simulink model "EV_Modeling_old"  (R2024b)
settings: Solver=FixedStepAuto  StartTime=0.0  StopTime=10382  FixedStep=0.1  RelTol=1e-3
values from neighbouring files (symbols this model uses):
  battery_SOC_SOC = battery_SOC(:,1)    [EV_Truck.m]    (also in simulink.m)
  battery_SOC_voltage = battery_SOC(:,2)    [EV_Truck.m]    (also in simulink.m)
  drag_coefficient_FV1 = table2array(drag_coefficient(:,3))    [simulink.m]
  drag_coefficient_FV2 = table2array(drag_coefficient(:,4))    [simulink.m]
  drag_coefficient_input = table2array(drag_coefficient(:,1))    [simulink.m]
  drag_coefficient_LV = table2array(drag_coefficient(:,2))    [simulink.m]
  electric_consumption_ressistancce = electric_consumption(:,2)    [EV_Truck.m]    (also in simulink.m)
  electric_consumption_voltage = electric_consumption(:,1)    [EV_Truck.m]    (also in simulink.m)
  motor_efficiency_efficiency = table2array(motor_efficiency(2:height(motor_efficiency),2:width(motor_efficiency)))    [EV_Truck.m]    (also in simulink.m)
  motor_efficiency_RPM = table2array(motor_efficiency(2:height(motor_efficiency),1))    [EV_Truck.m]    (also in simulink.m)
  motor_efficiency_torque = transpose(motor_efficiency_torque)    [EV_Truck.m]    (also in simulink.m)
  motor_RPM_torque = table2array(motor_torque(1:14,1))    [EV_Truck.m]    (also in simulink.m)
  motor_torque_RPM = table2array(motor_torque(1:14,2))    [EV_Truck.m]    (also in simulink.m)
undefined symbols (not defined in the file or in its folder): battery_builder_rtmsupport, battery_sli_rtmsupport, C1_mat, C2_mat, c_sqrt, DiscIntNeverNeededParam, dV0_mat, gcbh, n, Wc, Wm, x0
libraries: simulink x87, packLibrary_lib x30, nesl_utility x6, fl_lib x6, simulink_extras x3, mpcadaslib x2, slpidlib x1
(part 7 of 12)

== system EV_Modeling_old/LV/SOC Estimator (Kalman Filter)/Kalman Filter/UKBF 2RC ==
  CellVoltage : Inport
  Current : Inport  Port=2
  CellTemperature : Inport  Port=3
  InitialSOC : Inport  Port=4
  Constant : Constant  Value=chol(P0_2RC,'lower')
  Constant1 : Constant  Value=0  VectorParams1D=off
  Data Type Conversion{,1..3} (4 alike) : DataTypeConversion  OutDataTypeStr=double  SaturateOnIntegerOverflow=off  RndMeth=Floor
  Mux : Mux  Inputs=3
  Prediction-correction : Subsystem
  Reshape : Reshape  OutputDimensionality=Customize  OutputDimensions=[n,1]
  Reshape1 : Reshape
  Sigma points init : Subsystem
  xhat : Outport
  wires:
  Data Type Conversion/1 -> Prediction-correction/1(Current)
  Data Type Conversion3/1 -> Mux/1
  Data Type Conversion2/1 -> Prediction-correction/3(Voltage)
  Reshape/1 -> Sigma points init/1(x0)
  InitialSOC/1 -> Data Type Conversion3/1
  Constant/1 -> Sigma points init/2(A)
  Data Type Conversion1/1 -> Prediction-correction/2(Temperature)
  Constant1/1 -> Mux/3, Mux/2
  Prediction-correction/1(xhat) -> Reshape1/1
  Sigma points init/1(X0) -> Prediction-correction/4(X0)
  CellTemperature/1 -> Data Type Conversion1/1
  CellVoltage/1 -> Data Type Conversion2/1
  Mux/1 -> Reshape/1
  Current/1 -> Data Type Conversion/1
  Reshape1/1 -> xhat/1

== system EV_Modeling_old/LV/SOC Estimator (Kalman Filter)/Kalman Filter/UKF ==
  CellVoltage : Inport
  Current : Inport  Port=2
  CellTemperature : Inport  Port=3
  InitialSOC : Inport  Port=4
  Correction : Subsystem
  Delay - X : Subsystem
      settings: PortSchema="{\"entries\":[{\"content\":{\"sides\":[{\"content\":{\"connectorIds\":[\"In1\"]},\"type\":\"ConnectorPlacement.EquallySpacedRectSide\",\"uuid\":\"3362b6e3-9ef0-414f-8c36-2f543f704d9c\"},{\"content\":{\"connectorIds\":[\"Out1\",\"In2\"],\"side\":\"RIGHT\"},\"type\":\"ConnectorPlacement.EquallySpacedRectSide\",\"uuid\":\"11e7d0c5-4a27-4b8c-b505-ab30596c2b25\"},{\"content\":{\"connectorIds\":[],\"side\":\"TOP\"},\"type\":\"ConnectorPlacement.EquallySpacedRectSide\",\"uuid\":\"2d2b4d79-d4b9-4064-9377-c3a75a280e90\"}]},\"type\":\"ConnectorPlacement.EquallySpacedConnector\",\"uuid\":\"61e54eb8-002c-4ced-aad8-a34ad65d09af\"}],\"packageUris\":[\"http://schema.mathworks.com/mf0/Connector/R2020b\"],\"version\":\"1.0\"}"
  Prediction : Subsystem
  Rate Transition{,1..3} (4 alike) : RateTransition  OutPortSampleTime=Ts
  Reshape : Reshape
  Sigma points : Subsystem
  Sum : Sum  Inputs=+-|
  Unit Delay - P : UnitDelay  InitialCondition=chol(P0,'lower')  SampleTime=Ts  HasFrameUpgradeWarning=on
  xhat : Outport
  wires:
  Prediction/1(Yk1_k) -> Sum/2
  CellVoltage/1 -> Rate Transition/1
  Prediction/5(Pk1k) -> Correction/5(Pk1_k)
  Current/1 -> Rate Transition1/1
  Delay - X/1(y) -> Sigma points/1(x)
  Sum/1 -> Correction/1(Vt_error)
  Sigma points/1(X) -> Prediction/3(X)
  CellTemperature/1 -> Rate Transition2/1
  Prediction/4(Py) -> Correction/4(Py)
  Prediction/3(Pxy) -> Correction/3(Pxy)
  Unit Delay - P/1 -> Sigma points/2(P)
  Correction/1(xk1_k1) -> Delay - X/1(u), Reshape/1
  Correction/2(Pk1_k1) -> Unit Delay - P/1
  Prediction/2(Xk1_k) -> Correction/2(xk1_k)
  Reshape/1 -> xhat/1
  Rate Transition/1 -> Sum/1
  Rate Transition1/1 -> Prediction/1(Current)
  Rate Transition2/1 -> Prediction/2(Temperature)
  InitialSOC/1 -> Rate Transition3/1
  Rate Transition3/1 -> Delay - X/2(SOC0)

== system EV_Modeling_old/LV/SOC Estimator (Kalman Filter)/Kalman Filter/UKF 2RC ==
  CellVoltage : Inport
  Current : Inport  Port=2
  CellTemperature : Inport  Port=3
  InitialSOC : Inport  Port=4
  Correction : Subsystem
  Delay - X : Subsystem
      settings: PortSchema="{\"entries\":[{\"content\":{\"sides\":[{\"content\":{\"connectorIds\":[\"In1\"]},\"type\":\"ConnectorPlacement.EquallySpacedRectSide\",\"uuid\":\"3362b6e3-9ef0-414f-8c36-2f543f704d9c\"},{\"content\":{\"connectorIds\":[\"Out1\",\"In2\"],\"side\":\"RIGHT\"},\"type\":\"ConnectorPlacement.EquallySpacedRectSide\",\"uuid\":\"11e7d0c5-4a27-4b8c-b505-ab30596c2b25\"},{\"content\":{\"connectorIds\":[],\"side\":\"TOP\"},\"type\":\"ConnectorPlacement.EquallySpacedRectSide\",\"uuid\":\"2d2b4d79-d4b9-4064-9377-c3a75a280e90\"}]},\"type\":\"ConnectorPlacement.EquallySpacedConnector\",\"uuid\":\"61e54eb8-002c-4ced-aad8-a34ad65d09af\"}],\"packageUris\":[\"http://schema.mathworks.com/mf0/Connector/R2020b\"],\"version\":\"1.0\"}"
  Prediction : Subsystem
  Rate Transition{,1..3} (4 alike) : RateTransition  OutPortSampleTime=Ts
  Reshape : Reshape
  Sigma points : Subsystem
  Sum : Sum  Inputs=+-|
  Unit Delay - P : UnitDelay  InitialCondition=chol(P0_2RC,'lower')  SampleTime=Ts  HasFrameUpgradeWarning=on
  xhat : Outport
  wires:
  Rate Transition/1 -> Sum/1
  Rate Transition3/1 -> Delay - X/2(SOC0)
  CellTemperature/1 -> Rate Transition2/1
  Correction/1(xk1_k1) -> Delay - X/1(u), Reshape/1
  Prediction/2(Xk1_k) -> Correction/2(xk1_k)
  InitialSOC/1 -> Rate Transition3/1
  Unit Delay - P/1 -> Sigma points/2(P)
  Current/1 -> Rate Transition1/1
  Prediction/1(Yk1_k) -> Sum/2
  Rate Transition1/1 -> Prediction/1(Current)
  Rate Transition2/1 -> Prediction/2(Temperature)
  Sum/1 -> Correction/1(Vt_error)
  Prediction/5(Pk1k) -> Correction/5(Pk1_k)
  Prediction/4(Py) -> Correction/4(Py)
  Prediction/3(Pxy) -> Correction/3(Pxy)
  Sigma points/1(X) -> Prediction/3(X)
  Reshape/1 -> xhat/1
  CellVoltage/1 -> Rate Transition/1
  Correction/2(Pk1_k1) -> Unit Delay - P/1
  Delay - X/1(y) -> Sigma points/1(x)

== system EV_Modeling_old/LV/Subsystem/Pack1/ModuleAssembly1 ==
  note: Battery Modules
  note: Output Signals
  Module1 : packLibrary_lib/Modules/ModuleType1  SOC_vecCell=[0, .1, .25, .5, .75, .9, 1]  V0_vecCell=[3.5057, 3.566, 3.6337, 3.7127, 3.9259, 4.0777, 4.1928] V  V_rangeCell=[0, inf] V  R0_vecCell=[.0085, .0085, .0087, .0082, .0083, .0085, .0085] Ohm  AHCell=5 Ah  extrapolation_optionCell=simscape.enum.extrapolation.nearest  P=3  S=11  iCell_specify=off  iCell_priority=None  iCell=0 A  iCell_nominal_specify=off  iCell_nominal_value=1  iCell_nominal_unit=A  vCell_specify=off  vCell_priority=None  vCell=0 V  vCell_nominal_specify=off  vCell_nominal_value=1  vCell_nominal_unit=V  socCell_specify=off  socCell_priority=High  socCell=1  socCell_nominal_specify=off  socCell_nominal_value=1  socCell_nominal_unit=1  numCyclesCell_specify=off  numCyclesCell_priority=High  numCyclesCell=0  numCyclesCell_nominal_specify=off  numCyclesCell_nominal_value=1  numCyclesCell_nominal_unit=1  vParallelAssembly_specify=off  vParallelAssembly_priority=None  vParallelAssembly=repmat(0, 11, 1) V  vParallelAssembly_nominal_specify=off  vParallelAssembly_nominal_value=1  vParallelAssembly_nominal_unit=V  socParallelAssembly_specify=off  socParallelAssembly_priority=None  socParallelAssembly=repmat(1, 11, 1)  socParallelAssembly_nominal_specify=off  socParallelAssembly_nominal_value=1  socParallelAssembly_nominal_unit=1
      settings: InternalSimscapePortConfiguration="{\"Bottom\":[{\"id\":\"n\",\"label\":\"-\",\"type\":\"foundation.electrical.electrical\"}],\"Left\":[],\"Right\":[],\"Top\":[{\"id\":\"p\",\"label\":\"+\",\"type\":\"foundation.electrical.electrical\"}]}"
  Module1_outputs : SimscapeProbe  BoundBlock=553  Variables="{\"iCell\":{\"Unit\":\"A\",\"PortLabel\":\"iCell\",\"Probing\":\"ON\"},\"numCyclesCell\":{\"Unit\":\"1\",\"PortLabel\":\"numCyclesCell\",\"Probing\":\"ON\"},\"socCell\":{\"Unit\":\"1\",\"PortLabel\":\"socCell\",\"Probing\":\"ON\"},\"socParallelAssembly\":{\"Unit\":\"1\",\"PortLabel\":\"socParallelAssembly\",\"Probing\":\"ON\"},\"vCell\":{\"Unit\":\"V\",\"PortLabel\":\"vCell\",\"Probing\":\"ON\"},\"vParallelAssembly\":{\"Unit\":\"V\",\"PortLabel\":\"vParallelAssembly\",\"Probing\":\"ON\"}}"
  Module2 : packLibrary_lib/Modules/ModuleType1  SOC_vecCell=[0, .1, .25, .5, .75, .9, 1]  V0_vecCell=[3.5057, 3.566, 3.6337, 3.7127, 3.9259, 4.0777, 4.1928] V  V_rangeCell=[0, inf] V  R0_vecCell=[.0085, .0085, .0087, .0082, .0083, .0085, .0085] Ohm  AHCell=5 Ah  extrapolation_optionCell=simscape.enum.extrapolation.nearest  P=3  S=11  iCell_specify=off  iCell_priority=None  iCell=0 A  iCell_nominal_specify=off  iCell_nominal_value=1  iCell_nominal_unit=A  vCell_specify=off  vCell_priority=None  vCell=0 V  vCell_nominal_specify=off  vCell_nominal_value=1  vCell_nominal_unit=V  socCell_specify=off  socCell_priority=High  socCell=1  socCell_nominal_specify=off  socCell_nominal_value=1  socCell_nominal_unit=1  numCyclesCell_specify=off  numCyclesCell_priority=High  numCyclesCell=0  numCyclesCell_nominal_specify=off  numCyclesCell_nominal_value=1  numCyclesCell_nominal_unit=1  vParallelAssembly_specify=off  vParallelAssembly_priority=None  vParallelAssembly=repmat(0, 11, 1) V  vParallelAssembly_nominal_specify=off  vParallelAssembly_nominal_value=1  vParallelAssembly_nominal_unit=V  socParallelAssembly_specify=off  socParallelAssembly_priority=None  socParallelAssembly=repmat(1, 11, 1)  socParallelAssembly_nominal_specify=off  socParallelAssembly_nominal_value=1  socParallelAssembly_nominal_unit=1
      settings: InternalSimscapePortConfiguration="{\"Bottom\":[{\"id\":\"n\",\"label\":\"-\",\"type\":\"foundation.electrical.electrical\"}],\"Left\":[],\"Right\":[],\"Top\":[{\"id\":\"p\",\"label\":\"+\",\"type\":\"foundation.electrical.electrical\"}]}"
  Module2_outputs : SimscapeProbe  BoundBlock=555  Variables="{\"iCell\":{\"Unit\":\"A\",\"PortLabel\":\"iCell\",\"Probing\":\"ON\"},\"numCyclesCell\":{\"Unit\":\"1\",\"PortLabel\":\"numCyclesCell\",\"Probing\":\"ON\"},\"socCell\":{\"Unit\":\"1\",\"PortLabel\":\"socCell\",\"Probing\":\"ON\"},\"socParallelAssembly\":{\"Unit\":\"1\",\"PortLabel\":\"socParallelAssembly\",\"Probing\":\"ON\"},\"vCell\":{\"Unit\":\"V\",\"PortLabel\":\"vCell\",\"Probing\":\"ON\"},\"vParallelAssembly\":{\"Unit\":\"V\",\"PortLabel\":\"vParallelAssembly\",\"Probing\":\"ON\"}}"
  iCellMux : Mux  Inputs=2
  numCyclesCellMux : Mux  Inputs=2
  socCellMux : Mux  Inputs=2
  socParallelAssemblyMux : Mux  Inputs=2
  vCellMux : Mux  Inputs=2
  vParallelAssemblyMux : Mux  Inputs=2
  + : PMIOPort  Side=Left
  - : PMIOPort  Port=2  Side=Right
  iCell : Outport
  numCyclesCell : Outport  Port=2
  socCell : Outport  Port=3
  socParallelAssembly : Outport  Port=4
  vCell : Outport  Port=5
  vParallelAssembly : Outport  Port=6
  wires:
  Module1_outputs/1 -> [iCell1]
  iCellMux/1 -> iCell/1
  [iCell1] -> iCellMux/1
  Module1_outputs/2 -> [numCyclesCell1]
  numCyclesCellMux/1 -> numCyclesCell/1
  [numCyclesCell1] -> numCyclesCellMux/1
  Module1_outputs/3 -> [socCell1]
  socCellMux/1 -> socCell/1
  [socCell1] -> socCellMux/1
  Module1_outputs/4 -> [socParallelAssembly1]
  socParallelAssemblyMux/1 -> socParallelAssembly/1
  [socParallelAssembly1] -> socParallelAssemblyMux/1
  Module1_outputs/5 -> [vCell1]
  vCellMux/1 -> vCell/1
  [vCell1] -> vCellMux/1
  Module1_outputs/6 -> [vParallelAssembly1]
  vParallelAssemblyMux/1 -> vParallelAssembly/1
  [vParallelAssembly1] -> vParallelAssemblyMux/1
  Module2_outputs/1 -> [iCell2]
  [iCell2] -> iCellMux/2
  Module2_outputs/2 -> [numCyclesCell2]
  [numCyclesCell2] -> numCyclesCellMux/2
  Module2_outputs/3 -> [socCell2]
  [socCell2] -> socCellMux/2
  Module2_outputs/4 -> [socParallelAssembly2]
  [socParallelAssembly2] -> socParallelAssemblyMux/2
  Module2_outputs/5 -> [vCell2]
  [vCell2] -> vCellMux/2
  Module2_outputs/6 -> [vParallelAssembly2]
  [vParallelAssembly2] -> vParallelAssemblyMux/2
  connections:
  Module2/LConn1 -- Module1/RConn1
  Module1/LConn1 -- +/RConn1
  Module2/RConn1 -- -/RConn1

== system EV_Modeling_old/LV/Subsystem/Pack1/ModuleAssembly2 ==
  note: Battery Modules
  note: Output Signals
  Module1 : packLibrary_lib/Modules/ModuleType1  SOC_vecCell=[0, .1, .25, .5, .75, .9, 1]  V0_vecCell=[3.5057, 3.566, 3.6337, 3.7127, 3.9259, 4.0777, 4.1928] V  V_rangeCell=[0, inf] V  R0_vecCell=[.0085, .0085, .0087, .0082, .0083, .0085, .0085] Ohm  AHCell=5 Ah  extrapolation_optionCell=simscape.enum.extrapolation.nearest  P=3  S=11  iCell_specify=off  iCell_priority=None  iCell=0 A  iCell_nominal_specify=off  iCell_nominal_value=1  iCell_nominal_unit=A  vCell_specify=off  vCell_priority=None  vCell=0 V  vCell_nominal_specify=off  vCell_nominal_value=1  vCell_nominal_unit=V  socCell_specify=off  socCell_priority=High  socCell=1  socCell_nominal_specify=off  socCell_nominal_value=1  socCell_nominal_unit=1  numCyclesCell_specify=off  numCyclesCell_priority=High  numCyclesCell=0  numCyclesCell_nominal_specify=off  numCyclesCell_nominal_value=1  numCyclesCell_nominal_unit=1  vParallelAssembly_specify=off  vParallelAssembly_priority=None  vParallelAssembly=repmat(0, 11, 1) V  vParallelAssembly_nominal_specify=off  vParallelAssembly_nominal_value=1  vParallelAssembly_nominal_unit=V  socParallelAssembly_specify=off  socParallelAssembly_priority=None  socParallelAssembly=repmat(1, 11, 1)  socParallelAssembly_nominal_specify=off  socParallelAssembly_nominal_value=1  socParallelAssembly_nominal_unit=1
      settings: InternalSimscapePortConfiguration="{\"Bottom\":[{\"id\":\"n\",\"label\":\"-\",\"type\":\"foundation.electrical.electrical\"}],\"Left\":[],\"Right\":[],\"Top\":[{\"id\":\"p\",\"label\":\"+\",\"type\":\"foundation.electrical.electrical\"}]}"
  Module1_outputs : SimscapeProbe  BoundBlock=598  Variables="{\"iCell\":{\"Unit\":\"A\",\"PortLabel\":\"iCell\",\"Probing\":\"ON\"},\"numCyclesCell\":{\"Unit\":\"1\",\"PortLabel\":\"numCyclesCell\",\"Probing\":\"ON\"},\"socCell\":{\"Unit\":\"1\",\"PortLabel\":\"socCell\",\"Probing\":\"ON\"},\"socParallelAssembly\":{\"Unit\":\"1\",\"PortLabel\":\"socParallelAssembly\",\"Probing\":\"ON\"},\"vCell\":{\"Unit\":\"V\",\"PortLabel\":\"vCell\",\"Probing\":\"ON\"},\"vParallelAssembly\":{\"Unit\":\"V\",\"PortLabel\":\"vParallelAssembly\",\"Probing\":\"ON\"}}"
  Module2 : packLibrary_lib/Modules/ModuleType1  SOC_vecCell=[0, .1, .25, .5, .75, .9, 1]  V0_vecCell=[3.5057, 3.566, 3.6337, 3.7127, 3.9259, 4.0777, 4.1928] V  V_rangeCell=[0, inf] V  R0_vecCell=[.0085, .0085, .0087, .0082, .0083, .0085, .0085] Ohm  AHCell=5 Ah  extrapolation_optionCell=simscape.enum.extrapolation.nearest  P=3  S=11  iCell_specify=off  iCell_priority=None  iCell=0 A  iCell_nominal_specify=off  iCell_nominal_value=1  iCell_nominal_unit=A  vCell_specify=off  vCell_priority=None  vCell=0 V  vCell_nominal_specify=off  vCell_nominal_value=1  vCell_nominal_unit=V  socCell_specify=off  socCell_priority=High  socCell=1  socCell_nominal_specify=off  socCell_nominal_value=1  socCell_nominal_unit=1  numCyclesCell_specify=off  numCyclesCell_priority=High  numCyclesCell=0  numCyclesCell_nominal_specify=off  numCyclesCell_nominal_value=1  numCyclesCell_nominal_unit=1  vParallelAssembly_specify=off  vParallelAssembly_priority=None  vParallelAssembly=repmat(0, 11, 1) V  vParallelAssembly_nominal_specify=off  vParallelAssembly_nominal_value=1  vParallelAssembly_nominal_unit=V  socParallelAssembly_specify=off  socParallelAssembly_priority=None  socParallelAssembly=repmat(1, 11, 1)  socParallelAssembly_nominal_specify=off  socParallelAssembly_nominal_value=1  socParallelAssembly_nominal_unit=1
      settings: InternalSimscapePortConfiguration="{\"Bottom\":[{\"id\":\"n\",\"label\":\"-\",\"type\":\"foundation.electrical.electrical\"}],\"Left\":[],\"Right\":[],\"Top\":[{\"id\":\"p\",\"label\":\"+\",\"type\":\"foundation.electrical.electrical\"}]}"
  Module2_outputs : SimscapeProbe  BoundBlock=600  Variables="{\"iCell\":{\"Unit\":\"A\",\"PortLabel\":\"iCell\",\"Probing\":\"ON\"},\"numCyclesCell\":{\"Unit\":\"1\",\"PortLabel\":\"numCyclesCell\",\"Probing\":\"ON\"},\"socCell\":{\"Unit\":\"1\",\"PortLabel\":\"socCell\",\"Probing\":\"ON\"},\"socParallelAssembly\":{\"Unit\":\"1\",\"PortLabel\":\"socParallelAssembly\",\"Probing\":\"ON\"},\"vCell\":{\"Unit\":\"V\",\"PortLabel\":\"vCell\",\"Probing\":\"ON\"},\"vParallelAssembly\":{\"Unit\":\"V\",\"PortLabel\":\"vParallelAssembly\",\"Probing\":\"ON\"}}"
  iCellMux : Mux  Inputs=2
  numCyclesCellMux : Mux  Inputs=2
  socCellMux : Mux  Inputs=2
  socParallelAssemblyMux : Mux  Inputs=2
  vCellMux : Mux  Inputs=2
  vParallelAssemblyMux : Mux  Inputs=2
  + : PMIOPort  Side=Left
  - : PMIOPort  Port=2  Side=Right
  iCell : Outport
  numCyclesCell : Outport  Port=2
  socCell : Outport  Port=3
  socParallelAssembly : Outport  Port=4
  vCell : Outport  Port=5
  vParallelAssembly : Outport  Port=6
  wires:
  Module1_outputs/1 -> [iCell1]
  iCellMux/1 -> iCell/1
  [iCell1] -> iCellMux/1
  Module1_outputs/2 -> [numCyclesCell1]
  numCyclesCellMux/1 -> numCyclesCell/1
  [numCyclesCell1] -> numCyclesCellMux/1
  Module1_outputs/3 -> [socCell1]
  socCellMux/1 -> socCell/1
  [socCell1] -> socCellMux/1
  Module1_outputs/4 -> [socParallelAssembly1]
  socParallelAssemblyMux/1 -> socParallelAssembly/1
  [socParallelAssembly1] -> socParallelAssemblyMux/1
  Module1_outputs/5 -> [vCell1]
  vCellMux/1 -> vCell/1
  [vCell1] -> vCellMux/1
  Module1_outputs/6 -> [vParallelAssembly1]
  vParallelAssemblyMux/1 -> vParallelAssembly/1
  [vParallelAssembly1] -> vParallelAssemblyMux/1
  Module2_outputs/1 -> [iCell2]
  [iCell2] -> iCellMux/2
  Module2_outputs/2 -> [numCyclesCell2]
  [numCyclesCell2] -> numCyclesCellMux/2
  Module2_outputs/3 -> [socCell2]
  [socCell2] -> socCellMux/2
  Module2_outputs/4 -> [socParallelAssembly2]
  [socParallelAssembly2] -> socParallelAssemblyMux/2
  Module2_outputs/5 -> [vCell2]
  [vCell2] -> vCellMux/2
  Module2_outputs/6 -> [vParallelAssembly2]
  [vParallelAssembly2] -> vParallelAssemblyMux/2
  connections:
  Module2/LConn1 -- Module1/RConn1
  Module1/LConn1 -- +/RConn1
  Module2/RConn1 -- -/RConn1

== system EV_Modeling_old/LV/Subsystem/Pack1/ModuleAssembly3 ==
  note: Battery Modules
  note: Output Signals
  Module1 : packLibrary_lib/Modules/ModuleType1  SOC_vecCell=[0, .1, .25, .5, .75, .9, 1]  V0_vecCell=[3.5057, 3.566, 3.6337, 3.7127, 3.9259, 4.0777, 4.1928] V  V_rangeCell=[0, inf] V  R0_vecCell=[.0085, .0085, .0087, .0082, .0083, .0085, .0085] Ohm  AHCell=5 Ah  extrapolation_optionCell=simscape.enum.extrapolation.nearest  P=3  S=11  iCell_specify=off  iCell_priority=None  iCell=0 A  iCell_nominal_specify=off  iCell_nominal_value=1  iCell_nominal_unit=A  vCell_specify=off  vCell_priority=None  vCell=0 V  vCell_nominal_specify=off  vCell_nominal_value=1  vCell_nominal_unit=V  socCell_specify=off  socCell_priority=High  socCell=1  socCell_nominal_specify=off  socCell_nominal_value=1  socCell_nominal_unit=1  numCyclesCell_specify=off  numCyclesCell_priority=High  numCyclesCell=0  numCyclesCell_nominal_specify=off  numCyclesCell_nominal_value=1  numCyclesCell_nominal_unit=1  vParallelAssembly_specify=off  vParallelAssembly_priority=None  vParallelAssembly=repmat(0, 11, 1) V  vParallelAssembly_nominal_specify=off  vParallelAssembly_nominal_value=1  vParallelAssembly_nominal_unit=V  socParallelAssembly_specify=off  socParallelAssembly_priority=None  socParallelAssembly=repmat(1, 11, 1)  socParallelAssembly_nominal_specify=off  socParallelAssembly_nominal_value=1  socParallelAssembly_nominal_unit=1
      settings: InternalSimscapePortConfiguration="{\"Bottom\":[{\"id\":\"n\",\"label\":\"-\",\"type\":\"foundation.electrical.electrical\"}],\"Left\":[],\"Right\":[],\"Top\":[{\"id\":\"p\",\"label\":\"+\",\"type\":\"foundation.electrical.electrical\"}]}"
  Module1_outputs : SimscapeProbe  BoundBlock=643  Variables="{\"iCell\":{\"Unit\":\"A\",\"PortLabel\":\"iCell\",\"Probing\":\"ON\"},\"numCyclesCell\":{\"Unit\":\"1\",\"PortLabel\":\"numCyclesCell\",\"Probing\":\"ON\"},\"socCell\":{\"Unit\":\"1\",\"PortLabel\":\"socCell\",\"Probing\":\"ON\"},\"socParallelAssembly\":{\"Unit\":\"1\",\"PortLabel\":\"socParallelAssembly\",\"Probing\":\"ON\"},\"vCell\":{\"Unit\":\"V\",\"PortLabel\":\"vCell\",\"Probing\":\"ON\"},\"vParallelAssembly\":{\"Unit\":\"V\",\"PortLabel\":\"vParallelAssembly\",\"Probing\":\"ON\"}}"
  Module2 : packLibrary_lib/Modules/ModuleType1  SOC_vecCell=[0, .1, .25, .5, .75, .9, 1]  V0_vecCell=[3.5057, 3.566, 3.6337, 3.7127, 3.9259, 4.0777, 4.1928] V  V_rangeCell=[0, inf] V  R0_vecCell=[.0085, .0085, .0087, .0082, .0083, .0085, .0085] Ohm  AHCell=5 Ah  extrapolation_optionCell=simscape.enum.extrapolation.nearest  P=3  S=11  iCell_specify=off  iCell_priority=None  iCell=0 A  iCell_nominal_specify=off  iCell_nominal_value=1  iCell_nominal_unit=A  vCell_specify=off  vCell_priority=None  vCell=0 V  vCell_nominal_specify=off  vCell_nominal_value=1  vCell_nominal_unit=V  socCell_specify=off  socCell_priority=High  socCell=1  socCell_nominal_specify=off  socCell_nominal_value=1  socCell_nominal_unit=1  numCyclesCell_specify=off  numCyclesCell_priority=High  numCyclesCell=0  numCyclesCell_nominal_specify=off  numCyclesCell_nominal_value=1  numCyclesCell_nominal_unit=1  vParallelAssembly_specify=off  vParallelAssembly_priority=None  vParallelAssembly=repmat(0, 11, 1) V  vParallelAssembly_nominal_specify=off  vParallelAssembly_nominal_value=1  vParallelAssembly_nominal_unit=V  socParallelAssembly_specify=off  socParallelAssembly_priority=None  socParallelAssembly=repmat(1, 11, 1)  socParallelAssembly_nominal_specify=off  socParallelAssembly_nominal_value=1  socParallelAssembly_nominal_unit=1
      settings: InternalSimscapePortConfiguration="{\"Bottom\":[{\"id\":\"n\",\"label\":\"-\",\"type\":\"foundation.electrical.electrical\"}],\"Left\":[],\"Right\":[],\"Top\":[{\"id\":\"p\",\"label\":\"+\",\"type\":\"foundation.electrical.electrical\"}]}"
  Module2_outputs : SimscapeProbe  BoundBlock=645  Variables="{\"iCell\":{\"Unit\":\"A\",\"PortLabel\":\"iCell\",\"Probing\":\"ON\"},\"numCyclesCell\":{\"Unit\":\"1\",\"PortLabel\":\"numCyclesCell\",\"Probing\":\"ON\"},\"socCell\":{\"Unit\":\"1\",\"PortLabel\":\"socCell\",\"Probing\":\"ON\"},\"socParallelAssembly\":{\"Unit\":\"1\",\"PortLabel\":\"socParallelAssembly\",\"Probing\":\"ON\"},\"vCell\":{\"Unit\":\"V\",\"PortLabel\":\"vCell\",\"Probing\":\"ON\"},\"vParallelAssembly\":{\"Unit\":\"V\",\"PortLabel\":\"vParallelAssembly\",\"Probing\":\"ON\"}}"
  iCellMux : Mux  Inputs=2
  numCyclesCellMux : Mux  Inputs=2
  socCellMux : Mux  Inputs=2
  socParallelAssemblyMux : Mux  Inputs=2
  vCellMux : Mux  Inputs=2
  vParallelAssemblyMux : Mux  Inputs=2
  + : PMIOPort  Side=Left
  - : PMIOPort  Port=2  Side=Right
  iCell : Outport
  numCyclesCell : Outport  Port=2
  socCell : Outport  Port=3
  socParallelAssembly : Outport  Port=4
  vCell : Outport  Port=5
  vParallelAssembly : Outport  Port=6
  wires:
  Module1_outputs/1 -> [iCell1]
  iCellMux/1 -> iCell/1
  [iCell1] -> iCellMux/1
  Module1_outputs/2 -> [numCyclesCell1]
  numCyclesCellMux/1 -> numCyclesCell/1
  [numCyclesCell1] -> numCyclesCellMux/1
  Module1_outputs/3 -> [socCell1]
  socCellMux/1 -> socCell/1
  [socCell1] -> socCellMux/1
  Module1_outputs/4 -> [socParallelAssembly1]
  socParallelAssemblyMux/1 -> socParallelAssembly/1
  [socParallelAssembly1] -> socParallelAssemblyMux/1
  Module1_outputs/5 -> [vCell1]
  vCellMux/1 -> vCell/1
  [vCell1] -> vCellMux/1
  Module1_outputs/6 -> [vParallelAssembly1]
  vParallelAssemblyMux/1 -> vParallelAssembly/1
  [vParallelAssembly1] -> vParallelAssemblyMux/1
  Module2_outputs/1 -> [iCell2]
  [iCell2] -> iCellMux/2
  Module2_outputs/2 -> [numCyclesCell2]
  [numCyclesCell2] -> numCyclesCellMux/2
  Module2_outputs/3 -> [socCell2]
  [socCell2] -> socCellMux/2
  Module2_outputs/4 -> [socParallelAssembly2]
  [socParallelAssembly2] -> socParallelAssemblyMux/2
  Module2_outputs/5 -> [vCell2]
  [vCell2] -> vCellMux/2
  Module2_outputs/6 -> [vParallelAssembly2]
  [vParallelAssembly2] -> vParallelAssemblyMux/2
  connections:
  Module2/LConn1 -- Module1/RConn1
  Module1/LConn1 -- +/RConn1
  Module2/RConn1 -- -/RConn1

== system EV_Modeling_old/LV/Subsystem/Pack1/ModuleAssembly4 ==
  note: Battery Modules
  note: Output Signals
  Module1 : packLibrary_lib/Modules/ModuleType1  SOC_vecCell=[0, .1, .25, .5, .75, .9, 1]  V0_vecCell=[3.5057, 3.566, 3.6337, 3.7127, 3.9259, 4.0777, 4.1928] V  V_rangeCell=[0, inf] V  R0_vecCell=[.0085, .0085, .0087, .0082, .0083, .0085, .0085] Ohm  AHCell=5 Ah  extrapolation_optionCell=simscape.enum.extrapolation.nearest  P=3  S=11  iCell_specify=off  iCell_priority=None  iCell=0 A  iCell_nominal_specify=off  iCell_nominal_value=1  iCell_nominal_unit=A  vCell_specify=off  vCell_priority=None  vCell=0 V  vCell_nominal_specify=off  vCell_nominal_value=1  vCell_nominal_unit=V  socCell_specify=off  socCell_priority=High  socCell=1  socCell_nominal_specify=off  socCell_nominal_value=1  socCell_nominal_unit=1  numCyclesCell_specify=off  numCyclesCell_priority=High  numCyclesCell=0  numCyclesCell_nominal_specify=off  numCyclesCell_nominal_value=1  numCyclesCell_nominal_unit=1  vParallelAssembly_specify=off  vParallelAssembly_priority=None  vParallelAssembly=repmat(0, 11, 1) V  vParallelAssembly_nominal_specify=off  vParallelAssembly_nominal_value=1  vParallelAssembly_nominal_unit=V  socParallelAssembly_specify=off  socParallelAssembly_priority=None  socParallelAssembly=repmat(1, 11, 1)  socParallelAssembly_nominal_specify=off  socParallelAssembly_nominal_value=1  socParallelAssembly_nominal_unit=1
      settings: InternalSimscapePortConfiguration="{\"Bottom\":[{\"id\":\"n\",\"label\":\"-\",\"type\":\"foundation.electrical.electrical\"}],\"Left\":[],\"Right\":[],\"Top\":[{\"id\":\"p\",\"label\":\"+\",\"type\":\"foundation.electrical.electrical\"}]}"
  Module1_outputs : SimscapeProbe  BoundBlock=688  Variables="{\"iCell\":{\"Unit\":\"A\",\"PortLabel\":\"iCell\",\"Probing\":\"ON\"},\"numCyclesCell\":{\"Unit\":\"1\",\"PortLabel\":\"numCyclesCell\",\"Probing\":\"ON\"},\"socCell\":{\"Unit\":\"1\",\"PortLabel\":\"socCell\",\"Probing\":\"ON\"},\"socParallelAssembly\":{\"Unit\":\"1\",\"PortLabel\":\"socParallelAssembly\",\"Probing\":\"ON\"},\"vCell\":{\"Unit\":\"V\",\"PortLabel\":\"vCell\",\"Probing\":\"ON\"},\"vParallelAssembly\":{\"Unit\":\"V\",\"PortLabel\":\"vParallelAssembly\",\"Probing\":\"ON\"}}"
  Module2 : packLibrary_lib/Modules/ModuleType1  SOC_vecCell=[0, .1, .25, .5, .75, .9, 1]  V0_vecCell=[3.5057, 3.566, 3.6337, 3.7127, 3.9259, 4.0777, 4.1928] V  V_rangeCell=[0, inf] V  R0_vecCell=[.0085, .0085, .0087, .0082, .0083, .0085, .0085] Ohm  AHCell=5 Ah  extrapolation_optionCell=simscape.enum.extrapolation.nearest  P=3  S=11  iCell_specify=off  iCell_priority=None  iCell=0 A  iCell_nominal_specify=off  iCell_nominal_value=1  iCell_nominal_unit=A  vCell_specify=off  vCell_priority=None  vCell=0 V  vCell_nominal_specify=off  vCell_nominal_value=1  vCell_nominal_unit=V  socCell_specify=off  socCell_priority=High  socCell=1  socCell_nominal_specify=off  socCell_nominal_value=1  socCell_nominal_unit=1  numCyclesCell_specify=off  numCyclesCell_priority=High  numCyclesCell=0  numCyclesCell_nominal_specify=off  numCyclesCell_nominal_value=1  numCyclesCell_nominal_unit=1  vParallelAssembly_specify=off  vParallelAssembly_priority=None  vParallelAssembly=repmat(0, 11, 1) V  vParallelAssembly_nominal_specify=off  vParallelAssembly_nominal_value=1  vParallelAssembly_nominal_unit=V  socParallelAssembly_specify=off  socParallelAssembly_priority=None  socParallelAssembly=repmat(1, 11, 1)  socParallelAssembly_nominal_specify=off  socParallelAssembly_nominal_value=1  socParallelAssembly_nominal_unit=1
      settings: InternalSimscapePortConfiguration="{\"Bottom\":[{\"id\":\"n\",\"label\":\"-\",\"type\":\"foundation.electrical.electrical\"}],\"Left\":[],\"Right\":[],\"Top\":[{\"id\":\"p\",\"label\":\"+\",\"type\":\"foundation.electrical.electrical\"}]}"
  Module2_outputs : SimscapeProbe  BoundBlock=690  Variables="{\"iCell\":{\"Unit\":\"A\",\"PortLabel\":\"iCell\",\"Probing\":\"ON\"},\"numCyclesCell\":{\"Unit\":\"1\",\"PortLabel\":\"numCyclesCell\",\"Probing\":\"ON\"},\"socCell\":{\"Unit\":\"1\",\"PortLabel\":\"socCell\",\"Probing\":\"ON\"},\"socParallelAssembly\":{\"Unit\":\"1\",\"PortLabel\":\"socParallelAssembly\",\"Probing\":\"ON\"},\"vCell\":{\"Unit\":\"V\",\"PortLabel\":\"vCell\",\"Probing\":\"ON\"},\"vParallelAssembly\":{\"Unit\":\"V\",\"PortLabel\":\"vParallelAssembly\",\"Probing\":\"ON\"}}"
  iCellMux : Mux  Inputs=2
  numCyclesCellMux : Mux  Inputs=2
  socCellMux : Mux  Inputs=2
  socParallelAssemblyMux : Mux  Inputs=2
  vCellMux : Mux  Inputs=2
  vParallelAssemblyMux : Mux  Inputs=2
  + : PMIOPort  Side=Left
  - : PMIOPort  Port=2  Side=Right
  iCell : Outport
  numCyclesCell : Outport  Port=2
  socCell : Outport  Port=3
  socParallelAssembly : Outport  Port=4
  vCell : Outport  Port=5
  vParallelAssembly : Outport  Port=6
  wires:
  Module1_outputs/1 -> [iCell1]
  iCellMux/1 -> iCell/1
  [iCell1] -> iCellMux/1
  Module1_outputs/2 -> [numCyclesCell1]
  numCyclesCellMux/1 -> numCyclesCell/1
  [numCyclesCell1] -> numCyclesCellMux/1
  Module1_outputs/3 -> [socCell1]
  socCellMux/1 -> socCell/1
  [socCell1] -> socCellMux/1
  Module1_outputs/4 -> [socParallelAssembly1]
  socParallelAssemblyMux/1 -> socParallelAssembly/1
  [socParallelAssembly1] -> socParallelAssemblyMux/1
  Module1_outputs/5 -> [vCell1]
  vCellMux/1 -> vCell/1
  [vCell1] -> vCellMux/1
  Module1_outputs/6 -> [vParallelAssembly1]
  vParallelAssemblyMux/1 -> vParallelAssembly/1
  [vParallelAssembly1] -> vParallelAssemblyMux/1
  Module2_outputs/1 -> [iCell2]
  [iCell2] -> iCellMux/2
  Module2_outputs/2 -> [numCyclesCell2]
  [numCyclesCell2] -> numCyclesCellMux/2
  Module2_outputs/3 -> [socCell2]
  [socCell2] -> socCellMux/2
  Module2_outputs/4 -> [socParallelAssembly2]
  [socParallelAssembly2] -> socParallelAssemblyMux/2
  Module2_outputs/5 -> [vCell2]
  [vCell2] -> vCellMux/2
  Module2_outputs/6 -> [vParallelAssembly2]
  [vParallelAssembly2] -> vParallelAssemblyMux/2
  connections:
  Module2/LConn1 -- Module1/RConn1
  Module1/LConn1 -- +/RConn1
  Module2/RConn1 -- -/RConn1

== system EV_Modeling_old/LV/Subsystem/Pack1/ModuleAssembly5 ==
  note: Battery Modules
  note: Output Signals
  Module1 : packLibrary_lib/Modules/ModuleType1  SOC_vecCell=[0, .1, .25, .5, .75, .9, 1]  V0_vecCell=[3.5057, 3.566, 3.6337, 3.7127, 3.9259, 4.0777, 4.1928] V  V_rangeCell=[0, inf] V  R0_vecCell=[.0085, .0085, .0087, .0082, .0083, .0085, .0085] Ohm  AHCell=5 Ah  extrapolation_optionCell=simscape.enum.extrapolation.nearest  P=3  S=11  iCell_specify=off  iCell_priority=None  iCell=0 A  iCell_nominal_specify=off  iCell_nominal_value=1  iCell_nominal_unit=A  vCell_specify=off  vCell_priority=None  vCell=0 V  vCell_nominal_specify=off  vCell_nominal_value=1  vCell_nominal_unit=V  socCell_specify=off  socCell_priority=High  socCell=1  socCell_nominal_specify=off  socCell_nominal_value=1  socCell_nominal_unit=1  numCyclesCell_specify=off  numCyclesCell_priority=High  numCyclesCell=0  numCyclesCell_nominal_specify=off  numCyclesCell_nominal_value=1  numCyclesCell_nominal_unit=1  vParallelAssembly_specify=off  vParallelAssembly_priority=None  vParallelAssembly=repmat(0, 11, 1) V  vParallelAssembly_nominal_specify=off  vParallelAssembly_nominal_value=1  vParallelAssembly_nominal_unit=V  socParallelAssembly_specify=off  socParallelAssembly_priority=None  socParallelAssembly=repmat(1, 11, 1)  socParallelAssembly_nominal_specify=off  socParallelAssembly_nominal_value=1  socParallelAssembly_nominal_unit=1
      settings: InternalSimscapePortConfiguration="{\"Bottom\":[{\"id\":\"n\",\"label\":\"-\",\"type\":\"foundation.electrical.electrical\"}],\"Left\":[],\"Right\":[],\"Top\":[{\"id\":\"p\",\"label\":\"+\",\"type\":\"foundation.electrical.electrical\"}]}"
  Module1_outputs : SimscapeProbe  BoundBlock=733  Variables="{\"iCell\":{\"Unit\":\"A\",\"PortLabel\":\"iCell\",\"Probing\":\"ON\"},\"numCyclesCell\":{\"Unit\":\"1\",\"PortLabel\":\"numCyclesCell\",\"Probing\":\"ON\"},\"socCell\":{\"Unit\":\"1\",\"PortLabel\":\"socCell\",\"Probing\":\"ON\"},\"socParallelAssembly\":{\"Unit\":\"1\",\"PortLabel\":\"socParallelAssembly\",\"Probing\":\"ON\"},\"vCell\":{\"Unit\":\"V\",\"PortLabel\":\"vCell\",\"Probing\":\"ON\"},\"vParallelAssembly\":{\"Unit\":\"V\",\"PortLabel\":\"vParallelAssembly\",\"Probing\":\"ON\"}}"
  Module2 : packLibrary_lib/Modules/ModuleType1  SOC_vecCell=[0, .1, .25, .5, .75, .9, 1]  V0_vecCell=[3.5057, 3.566, 3.6337, 3.7127, 3.9259, 4.0777, 4.1928] V  V_rangeCell=[0, inf] V  R0_vecCell=[.0085, .0085, .0087, .0082, .0083, .0085, .0085] Ohm  AHCell=5 Ah  extrapolation_optionCell=simscape.enum.extrapolation.nearest  P=3  S=11  iCell_specify=off  iCell_priority=None  iCell=0 A  iCell_nominal_specify=off  iCell_nominal_value=1  iCell_nominal_unit=A  vCell_specify=off  vCell_priority=None  vCell=0 V  vCell_nominal_specify=off  vCell_nominal_value=1  vCell_nominal_unit=V  socCell_specify=off  socCell_priority=High  socCell=1  socCell_nominal_specify=off  socCell_nominal_value=1  socCell_nominal_unit=1  numCyclesCell_specify=off  numCyclesCell_priority=High  numCyclesCell=0  numCyclesCell_nominal_specify=off  numCyclesCell_nominal_value=1  numCyclesCell_nominal_unit=1  vParallelAssembly_specify=off  vParallelAssembly_priority=None  vParallelAssembly=repmat(0, 11, 1) V  vParallelAssembly_nominal_specify=off  vParallelAssembly_nominal_value=1  vParallelAssembly_nominal_unit=V  socParallelAssembly_specify=off  socParallelAssembly_priority=None  socParallelAssembly=repmat(1, 11, 1)  socParallelAssembly_nominal_specify=off  socParallelAssembly_nominal_value=1  socParallelAssembly_nominal_unit=1
      settings: InternalSimscapePortConfiguration="{\"Bottom\":[{\"id\":\"n\",\"label\":\"-\",\"type\":\"foundation.electrical.electrical\"}],\"Left\":[],\"Right\":[],\"Top\":[{\"id\":\"p\",\"label\":\"+\",\"type\":\"foundation.electrical.electrical\"}]}"
  Module2_outputs : SimscapeProbe  BoundBlock=735  Variables="{\"iCell\":{\"Unit\":\"A\",\"PortLabel\":\"iCell\",\"Probing\":\"ON\"},\"numCyclesCell\":{\"Unit\":\"1\",\"PortLabel\":\"numCyclesCell\",\"Probing\":\"ON\"},\"socCell\":{\"Unit\":\"1\",\"PortLabel\":\"socCell\",\"Probing\":\"ON\"},\"socParallelAssembly\":{\"Unit\":\"1\",\"PortLabel\":\"socParallelAssembly\",\"Probing\":\"ON\"},\"vCell\":{\"Unit\":\"V\",\"PortLabel\":\"vCell\",\"Probing\":\"ON\"},\"vParallelAssembly\":{\"Unit\":\"V\",\"PortLabel\":\"vParallelAssembly\",\"Probing\":\"ON\"}}"
  iCellMux : Mux  Inputs=2
  numCyclesCellMux : Mux  Inputs=2
  socCellMux : Mux  Inputs=2
  socParallelAssemblyMux : Mux  Inputs=2
  vCellMux : Mux  Inputs=2
  vParallelAssemblyMux : Mux  Inputs=2
  + : PMIOPort  Side=Left
  - : PMIOPort  Port=2  Side=Right
  iCell : Outport
  numCyclesCell : Outport  Port=2
  socCell : Outport  Port=3
  socParallelAssembly : Outport  Port=4
  vCell : Outport  Port=5
  vParallelAssembly : Outport  Port=6
  wires:
  Module1_outputs/1 -> [iCell1]
  iCellMux/1 -> iCell/1
  [iCell1] -> iCellMux/1
  Module1_outputs/2 -> [numCyclesCell1]
  numCyclesCellMux/1 -> numCyclesCell/1
  [numCyclesCell1] -> numCyclesCellMux/1
  Module1_outputs/3 -> [socCell1]
  socCellMux/1 -> socCell/1
  [socCell1] -> socCellMux/1
  Module1_outputs/4 -> [socParallelAssembly1]
  socParallelAssemblyMux/1 -> socParallelAssembly/1
  [socParallelAssembly1] -> socParallelAssemblyMux/1
  Module1_outputs/5 -> [vCell1]
  vCellMux/1 -> vCell/1
  [vCell1] -> vCellMux/1
  Module1_outputs/6 -> [vParallelAssembly1]
  vParallelAssemblyMux/1 -> vParallelAssembly/1
  [vParallelAssembly1] -> vParallelAssemblyMux/1
  Module2_outputs/1 -> [iCell2]
  [iCell2] -> iCellMux/2
  Module2_outputs/2 -> [numCyclesCell2]
  [numCyclesCell2] -> numCyclesCellMux/2
  Module2_outputs/3 -> [socCell2]
  [socCell2] -> socCellMux/2
  Module2_outputs/4 -> [socParallelAssembly2]
  [socParallelAssembly2] -> socParallelAssemblyMux/2
  Module2_outputs/5 -> [vCell2]
  [vCell2] -> vCellMux/2
  Module2_outputs/6 -> [vParallelAssembly2]
  [vParallelAssembly2] -> vParallelAssemblyMux/2
  connections:
  Module2/LConn1 -- Module1/RConn1
  Module1/LConn1 -- +/RConn1
  Module2/RConn1 -- -/RConn1

== system EV_Modeling_old/FV1/SOC Estimator (Kalman Filter)1/Kalman Filter/EKBF/Jacobian ==
  current : Inport
  Temperature : Inport  Port=2
  x : Inport  Port=3
  2-D Lookup Table C1 : Lookup_n-D  BreakpointsForDimension1=SOC_vec  BreakpointsForDimension2=T_vec  Table=C1_mat  InternalRulePriority=Speed  RndMeth=Simplest
      settings: InputPortMap=u0,u1
  2-D Lookup Table R0 : Lookup_n-D  BreakpointsForDimension1=SOC_vec  BreakpointsForDimension2=T_vec  Table=R0_mat  InternalRulePriority=Speed  RndMeth=Simplest
      settings: InputPortMap=u0,u1
  2-D Lookup Table R1 : Lookup_n-D  BreakpointsForDimension1=SOC_vec  BreakpointsForDimension2=T_vec  Table=R1_mat  InternalRulePriority=Speed  RndMeth=Simplest
      settings: InputPortMap=u0,u1
  2-D Lookup Table V0 : Lookup_n-D  BreakpointsForDimension1=SOC_vec  BreakpointsForDimension2=T_vec  Table=V0_mat  InternalRulePriority=Speed  RndMeth=Simplest
      settings: InputPortMap=u0,u1
  2-D Lookup Table dV0 : Lookup_n-D  BreakpointsForDimension1=SOC_vec  BreakpointsForDimension2=T_vec  Table=dV0_mat  InternalRulePriority=Speed  RndMeth=Simplest
      settings: InputPortMap=u0,u1
  Add1 : Sum  Inputs=-+
  Assignment : Assignment  NumberOfDimensions=2  DiagnosticForDimensions=Warning  IndexOptions=Index vector (dialog),Index vector (dialog)  Indices=2,2  OutputSizes=1,1
  Constant : Constant  Value=|
      | [0 0;
      | 0 0]
  Constant3 : Constant  Value=-1
  Constant4 : Constant  Value=-1
  Divide1 : Product  Inputs=*/
  Divide2 : Product  Inputs=/*
  Gain : Gain  Gain=-1/(AH*3600)
  Mux : Mux  Inputs=2
  Mux1 : Mux  Inputs=2
  Product : Product
  Product2 : Product  Inputs=/*
  Product6 : Product
  Selector : Selector  InputPortWidth=2  IndexOptions=Index vector (dialog)  Indices=1  OutputSizes=1
  Selector1 : Selector  InputPortWidth=2  IndexOptions=Index vector (dialog)  Indices=2  OutputSizes=1
  Sum2 : Sum  Inputs=+--
  Transpose1 : Math  Operator=transpose
  Vt_model : Outport
  f(x) : Outport  Port=2
  F : Outport  Port=3
  H : Outport  Port=4
  wires:
  Product/1 -> Product2/1, Divide2/1  "tau1"
  2-D Lookup Table V0/1 -> Sum2/1  "V0"
  Sum2/1 -> Vt_model/1
  Selector1/1 -> Sum2/3, Divide2/2  "V1"
  Product6/1 -> Sum2/2
  2-D Lookup Table R0/1 -> Product6/1  "R0"
  Constant3/1 -> Product2/2
  Assignment/1 -> F/1
  Product2/1 -> Assignment/2
  Constant/1 -> Assignment/1
  Selector/1 -> 2-D Lookup Table C1/1, 2-D Lookup Table dV0/1, 2-D Lookup Table V0/1, 2-D Lookup Table R0/1, 2-D Lookup Table R1/1  "SOC"
  Temperature/1 -> 2-D Lookup Table dV0/2, 2-D Lookup Table V0/2, 2-D Lookup Table R0/2, 2-D Lookup Table C1/2, 2-D Lookup Table R1/2
  x/1 -> Selector1/1, Selector/1
  Mux1/1 -> Transpose1/1
  Transpose1/1 -> H/1
  Constant4/1 -> Mux1/2
  2-D Lookup Table dV0/1 -> Mux1/1  "dV0"
  Divide1/1 -> Add1/2  "Current/C1"
  Mux/1 -> f(x)/1
  2-D Lookup Table C1/1 -> Divide1/2, Product/2  "C1"
  2-D Lookup Table R1/1 -> Product/1  "R1"
  Add1/1 -> Mux/2
  current/1 -> Product6/2, Gain/1, Divide1/1  "Current"
  Gain/1 -> Mux/1
  Divide2/1 -> Add1/1

== system EV_Modeling_old/FV1/SOC Estimator (Kalman Filter)1/Kalman Filter/EKBF/Prediction-correction ==
  f(x) : Inport
  F : Inport  Port=2
  H : Inport  Port=3
  InitialSOC : Inport  Port=4
  Vt_error : Inport  Port=5
  Constant : Constant  Value=Q
  Constant1 : Constant  Value=double(R)
  Constant2 : Constant  Value=eye(size(R,1))
  Constant3 : Constant  Value=0
  Divide : Product  Inputs=*/  Multiplication=Matrix(*)
  Integrator : Integrator  InitialCondition=double(P0)
  Integrator1 : Integrator  InitialConditionSource=external  InitialCondition=x0
  Mux : Mux  Inputs=2
  Product : Product  Multiplication=Matrix(*)
  Product3 : Product  Multiplication=Matrix(*)
  Product4 : Product  Inputs=3  Multiplication=Matrix(*)
  Product5 : Product  Inputs=3  Multiplication=Matrix(*)
  Product6 : Product  Multiplication=Matrix(*)
  Reshape : Reshape  OutputDimensionality=Customize  OutputDimensions=[n,1]
  Sum : Sum  Inputs=++-+
  Sum2 : Sum  Inputs=|++
  Transpose : Math  Operator=transpose
  Transpose1 : Math  Operator=transpose
  x : Outport
  wires:
  f(x)/1 -> Sum2/1
  Sum2/1 -> Integrator1/1
  Product6/1 -> Sum2/2
  Vt_error/1 -> Product6/2
  H/1 -> Product4/2, Transpose1/1
  F/1 -> Transpose/1, Product/1
  Integrator1/1 -> x/1
  Product5/1 -> Product6/1, Product4/1
  Constant2/1 -> Divide/1
  Divide/1 -> Product5/3
  Constant1/1 -> Divide/2
  Transpose1/1 -> Product5/2
  Sum/1 -> Integrator/1  "Pdot"
  Constant/1 -> Sum/4
  Product4/1 -> Sum/3
  Transpose/1 -> Product3/2
  Product3/1 -> Sum/2
  Product/1 -> Sum/1
  Integrator/1 -> Product5/1, Product4/3, Product/2, Product3/1
  Mux/1 -> Reshape/1
  InitialSOC/1 -> Mux/1
  Constant3/1 -> Mux/2
  Reshape/1 -> Integrator1/2

== system EV_Modeling_old/FV1/SOC Estimator (Kalman Filter)1/Kalman Filter/EKBF 2RC/Jacobian ==
  current : Inport
  Temperature : Inport  Port=2
  x : Inport  Port=3
  2-D Lookup Table C1 : Lookup_n-D  BreakpointsForDimension1=SOC_vec  BreakpointsForDimension2=T_vec  Table=C1_mat  InternalRulePriority=Speed  RndMeth=Simplest
      settings: InputPortMap=u0,u1
  2-D Lookup Table C2 : Lookup_n-D  BreakpointsForDimension1=SOC_vec  BreakpointsForDimension2=T_vec  Table=C2_mat  InternalRulePriority=Speed  RndMeth=Simplest
      settings: InputPortMap=u0,u1
  2-D Lookup Table R0 : Lookup_n-D  BreakpointsForDimension1=SOC_vec  BreakpointsForDimension2=T_vec  Table=R0_mat  InternalRulePriority=Speed  RndMeth=Simplest
      settings: InputPortMap=u0,u1
  2-D Lookup Table R1 : Lookup_n-D  BreakpointsForDimension1=SOC_vec  BreakpointsForDimension2=T_vec  Table=R1_mat  InternalRulePriority=Speed  RndMeth=Simplest
      settings: InputPortMap=u0,u1
  2-D Lookup Table R2 : Lookup_n-D  BreakpointsForDimension1=SOC_vec  BreakpointsForDimension2=T_vec  Table=R2_mat  InternalRulePriority=Speed  RndMeth=Simplest
      settings: InputPortMap=u0,u1
  2-D Lookup Table V0 : Lookup_n-D  BreakpointsForDimension1=SOC_vec  BreakpointsForDimension2=T_vec  Table=V0_mat  InternalRulePriority=Speed  RndMeth=Simplest
      settings: InputPortMap=u0,u1
  2-D Lookup Table dV0 : Lookup_n-D  BreakpointsForDimension1=SOC_vec  BreakpointsForDimension2=T_vec  Table=dV0_mat  InternalRulePriority=Speed  RndMeth=Simplest
      settings: InputPortMap=u0,u1
  Add1 : Sum  Inputs=-+
  Add2 : Sum  Inputs=-+
  Assignment : Assignment  NumberOfDimensions=2  DiagnosticForDimensions=Warning  IndexOptions=Index vector (dialog),Index vector (dialog)  Indices=2,2  OutputSizes=1,1
  Assignment1 : Assignment  NumberOfDimensions=2  DiagnosticForDimensions=Warning  IndexOptions=Index vector (dialog),Index vector (dialog)  Indices=3,3  OutputSizes=1,1
  Constant : Constant  Value=|
      | [0 0 0;
      | 0 0 0;0 0 0]
  Constant3 : Constant  Value=-1
  Constant4 : Constant  Value=-1
  Divide1 : Product  Inputs=*/
  Divide2 : Product  Inputs=/*
  Divide3 : Product  Inputs=/*
  Divide4 : Product  Inputs=*/
  Gain : Gain  Gain=-1/(AH*3600)
  Mux : Mux  Inputs=3
  Mux1 : Mux  Inputs=3
  Product : Product
  Product2 : Product  Inputs=/*
  Product3 : Product
  Product4 : Product  Inputs=*/
  Product6 : Product
  Selector : Selector  InputPortWidth=3  IndexOptions=Index vector (dialog)  Indices=1  OutputSizes=1
  Selector2 : Selector  InputPortWidth=3  IndexOptions=Index vector (dialog)  Indices=2  OutputSizes=1
  Selector3 : Selector  InputPortWidth=3  IndexOptions=Index vector (dialog)  Indices=3  OutputSizes=1
  Sum : Sum
  Sum2 : Sum  Inputs=+--
  Transpose1 : Math  Operator=transpose
  Vt_model : Outport
  f(x) : Outport  Port=2
  F : Outport  Port=3
  H : Outport  Port=4
  wires:
  Divide4/1 -> Add2/2  "Current/C2"
  Add2/1 -> Mux/3
  Divide3/1 -> Add2/1
  Selector3/1 -> Sum/2, Divide3/2  "V2"
  Selector2/1 -> Sum/1, Divide2/2  "V1"
  Sum/1 -> Sum2/3  "V1+V2"
  Product4/1 -> Assignment1/2
  Product3/1 -> Product4/2, Divide3/1  "tau2"
  2-D Lookup Table C2/1 -> Divide4/2, Product3/2
  2-D Lookup Table R2/1 -> Product3/1
  Assignment1/1 -> F/1
  Assignment/1 -> Assignment1/1
  Product/1 -> Product2/1, Divide2/1  "tau1"
  2-D Lookup Table V0/1 -> Sum2/1  "V0"
  Sum2/1 -> Vt_model/1
  Product6/1 -> Sum2/2
  2-D Lookup Table R0/1 -> Product6/1  "R0"
  Constant3/1 -> Product4/1, Product2/2
  Product2/1 -> Assignment/2
  Constant/1 -> Assignment/1
  Selector/1 -> 2-D Lookup Table C1/1, 2-D Lookup Table dV0/1, 2-D Lookup Table V0/1, 2-D Lookup Table R0/1, 2-D Lookup Table C2/1, 2-D Lookup Table R2/1, 2-D Lookup Table R1/1  "SOC"
  Temperature/1 -> 2-D Lookup Table dV0/2, 2-D Lookup Table V0/2, 2-D Lookup Table R0/2, 2-D Lookup Table C2/2, 2-D Lookup Table R2/2, 2-D Lookup Table C1/2, 2-D Lookup Table R1/2
  x/1 -> Selector2/1, Selector3/1, Selector/1
  Mux1/1 -> Transpose1/1
  Transpose1/1 -> H/1
  Constant4/1 -> Mux1/2, Mux1/3
  2-D Lookup Table dV0/1 -> Mux1/1  "dV0"
  Divide1/1 -> Add1/2  "Current/C1"
  Mux/1 -> f(x)/1
  2-D Lookup Table C1/1 -> Divide1/2, Product/2  "C1"
  2-D Lookup Table R1/1 -> Product/1  "R1"
  Add1/1 -> Mux/2
  current/1 -> Product6/2, Gain/1, Divide1/1, Divide4/1  "Current"
  Gain/1 -> Mux/1
  Divide2/1 -> Add1/1

== system EV_Modeling_old/FV1/SOC Estimator (Kalman Filter)1/Kalman Filter/EKBF 2RC/Prediction-correction ==
  f(x) : Inport
  F : Inport  Port=2
  H : Inport  Port=3
  InitialSOC : Inport  Port=4
  Vt_error : Inport  Port=5
  Constant : Constant  Value=Q_2RC
  Constant1 : Constant  Value=double(R)
  Constant2 : Constant  Value=eye(size(R,1))
  Constant3 : Constant  Value=0
  Divide : Product  Inputs=*/  Multiplication=Matrix(*)
  Integrator : Integrator  InitialCondition=double(P0_2RC)
  Integrator1 : Integrator  InitialConditionSource=external  InitialCondition=x0
  Mux : Mux  Inputs=3
  Product : Product  Multiplication=Matrix(*)
  Product3 : Product  Multiplication=Matrix(*)
  Product4 : Product  Inputs=3  Multiplication=Matrix(*)
  Product5 : Product  Inputs=3  Multiplication=Matrix(*)
  Product6 : Product  Multiplication=Matrix(*)
  Sum : Sum  Inputs=++-+
  Sum2 : Sum  Inputs=|++
  Transpose : Math  Operator=transpose
  Transpose1 : Math  Operator=transpose
  x : Outport
  wires:
  Constant3/1 -> Mux/2, Mux/3
  Constant2/1 -> Divide/1
  Constant1/1 -> Divide/2
  Constant/1 -> Sum/4
  InitialSOC/1 -> Mux/1
  Mux/1 -> Integrator1/2
  Integrator/1 -> Product3/1, Product/2, Product4/3, Product5/1
  Product/1 -> Sum/1
  Product3/1 -> Sum/2
  Transpose/1 -> Product3/2
  Product4/1 -> Sum/3
  Sum/1 -> Integrator/1  "Pdot"
  Transpose1/1 -> Product5/2
  Divide/1 -> Product5/3
  Product5/1 -> Product4/1, Product6/1
  Integrator1/1 -> x/1
  F/1 -> Product/1, Transpose/1
  H/1 -> Transpose1/1, Product4/2
  Vt_error/1 -> Product6/2
  Product6/1 -> Sum2/2
  Sum2/1 -> Integrator1/1
  f(x)/1 -> Sum2/1

== system EV_Modeling_old/FV1/SOC Estimator (Kalman Filter)1/Kalman Filter/EKF/Correction ==
  Vt_error : Inport
  H : Inport  Port=2
  xk1_k : Inport  Port=3
  Pk1_k : Inport  Port=4
  Constant : Constant  Value=R
  Constant1 : Constant  Value=eye(size(R,1))
  Constant2 : Constant  Value=eye(size(Q,1))  OutDataTypeStr=Inherit: Inherit via back propagation
  Data Type Conversion Inherited : simulink/Signal Attributes/Data Type Conversion Inherited  ConvertRealWorld=Real World Value  DoSatur=off
  Data Type Conversion Inherited1 : simulink/Signal Attributes/Data Type Conversion Inherited  ConvertRealWorld=Real World Value  DoSatur=off
  Divide : Product  Inputs=*/  Multiplication=Matrix(*)
  Product{,1,3..5} (5 alike) : Product  Multiplication=Matrix(*)
  Product2 : Product  Inputs=3  Multiplication=Matrix(*)
  Sum : Sum  Inputs=++|
  Sum2 : Sum  Inputs=|++
  Sum3 : Sum  Inputs=-+|
  Transpose : Math  Operator=transpose
  xk1_k1 : Outport
  Pk1_k1 : Outport  Port=2
  wires:
  H/1 -> Product4/2, Product2/1, Transpose/1
  Transpose/1 -> Product2/3, Product/2
  Pk1_k/1 -> Product5/2, Product2/2, Product/1
  Product/1 -> Data Type Conversion Inherited1/1, Product1/1
  Product2/1 -> Sum2/1
  Constant/1 -> Sum2/2
  Product1/1 -> Product4/1, Product3/1  "Kk1"
  Sum2/1 -> Divide/2
  Divide/1 -> Product1/2
  xk1_k/1 -> Sum/2
  Vt_error/1 -> Product3/2
  Product3/1 -> Sum/1
  Sum/1 -> xk1_k1/1
  Product4/1 -> Data Type Conversion Inherited/1, Sum3/1
  Sum3/1 -> Product5/1
  Product5/1 -> Pk1_k1/1
  Data Type Conversion Inherited/1 -> Sum3/2
  Constant2/1 -> Data Type Conversion Inherited/2
  Data Type Conversion Inherited1/1 -> Divide/1
  Constant1/1 -> Data Type Conversion Inherited1/2
